simulink model "idc2ff_digital"  (Simulink 8.6)
settings: Solver=ode45  StartTime=0.0  StopTime=10.0  RelTol=1e-3
undefined symbols (not defined in the file or in its folder): M, OSR, tclk
settings Model: Creator=chench  LastModifiedBy=derek
settings OptimizationCC: InitFltsAndDblsToZero=on
settings DebuggingCC: SaveWithParameterizedLinksMsg=none  SignalResolutionControl=TryResolveAllWithWarning  MultiTaskDSMMsg=warning  MultiTaskCondExecSysMsg=none  FcnCallInpInsideContextMsg=UseLocalSettings
settings GRTTargetCC: TargetFcnLib=ansi_tfl_tmw.mat

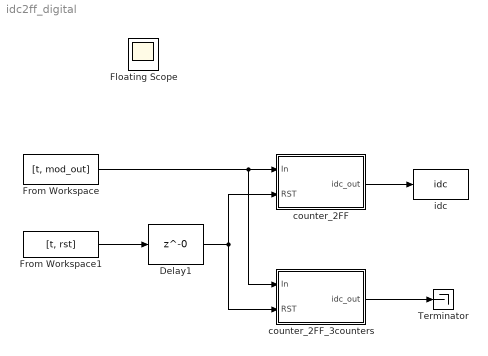
== system idc2ff_digital ==
  Delay1 : Delay  DelayLength=0  InitialCondition=0  InputProcessing=Inherited
  From Workspace : FromWorkspace  VariableName=[t, mod_out]  SampleTime=tclk  Interpolate=off  OutputAfterFinalValue=Holding final value
  From Workspace1 : FromWorkspace  VariableName=[t, rst]  SampleTime=tclk  Interpolate=off  OutputAfterFinalValue=Holding final value
  Terminator : Terminator
  counter_2FF : Subsystem
  counter_2FF_3counters : Subsystem
  idc : ToWorkspace  VariableName=idc  SampleTime=-1
  Floating Scope : Scope
  wires:
  From Workspace/1 -> counter_2FF/1(In), counter_2FF_3counters/1(In)
  counter_2FF/1(idc_out) -> idc/1
  From Workspace1/1 -> Delay1/1
  Delay1/1 -> counter_2FF/2(RST), counter_2FF_3counters/2(RST)
  counter_2FF_3counters/1(idc_out) -> Terminator/1

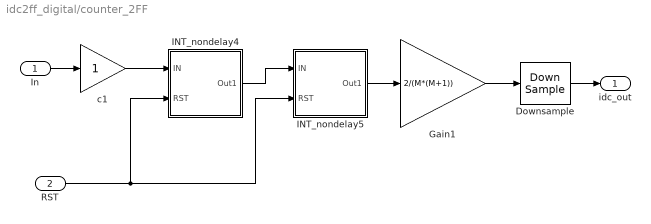
== system idc2ff_digital/counter_2FF ==
  In : Inport
  RST : Inport  Port=2
  Downsample : DownSample  N=OSR  phase=OSR-1  RateOptions=Allow multirate processing
  Gain1 : Gain  Gain=2/(M*(M+1))
  INT_nondelay4 : Subsystem
  INT_nondelay5 : Subsystem
  c1 : Gain  SaturateOnIntegerOverflow=on  OutDataTypeStr=Inherit: Same as input  ParamDataTypeStr=Inherit: Same as input
  idc_out : Outport
  wires:
  RST/1 -> INT_nondelay5/2(RST), INT_nondelay4/2(RST)
  Downsample/1 -> idc_out/1
  c1/1 -> INT_nondelay4/1(IN)
  In/1 -> c1/1
  INT_nondelay4/1(Out1) -> INT_nondelay5/1(IN)
  Gain1/1 -> Downsample/1
  INT_nondelay5/1(Out1) -> Gain1/1

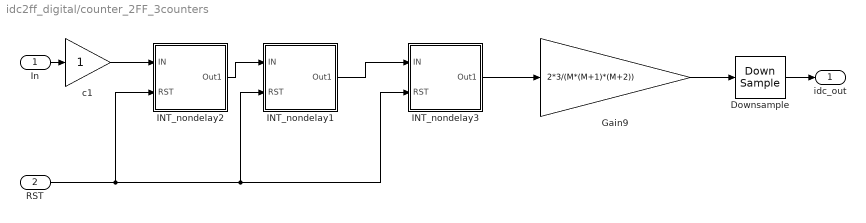
== system idc2ff_digital/counter_2FF_3counters ==
  In : Inport
  RST : Inport  Port=2
  Downsample : DownSample  N=OSR  phase=OSR-1  RateOptions=Allow multirate processing
  Gain9 : Gain  Gain=2*3/(M*(M+1)*(M+2))
  INT_nondelay1 : Subsystem
  INT_nondelay2 : Subsystem
  INT_nondelay3 : Subsystem
  c1 : Gain  SaturateOnIntegerOverflow=on  OutDataTypeStr=Inherit: Same as input  ParamDataTypeStr=Inherit: Same as input
  idc_out : Outport
  wires:
  RST/1 -> INT_nondelay3/2(RST), INT_nondelay1/2(RST), INT_nondelay2/2(RST)
  Downsample/1 -> idc_out/1
  c1/1 -> INT_nondelay2/1(IN)
  In/1 -> c1/1
  INT_nondelay2/1(Out1) -> INT_nondelay1/1(IN)
  INT_nondelay1/1(Out1) -> INT_nondelay3/1(IN)
  INT_nondelay3/1(Out1) -> Gain9/1
  Gain9/1 -> Downsample/1

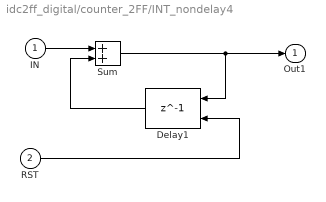
== system idc2ff_digital/counter_2FF/INT_nondelay4 ==
  IN : Inport
  RST : Inport  Port=2
  Delay1 : Delay  DelayLength=1  InitialCondition=0  ExternalReset=Rising  InputProcessing=Inherited
      settings: InputPortMap=u0,r5
  Sum : Sum  SaturateOnIntegerOverflow=on  InputSameDT=on  OutDataTypeStr=Inherit: Same as first input
  Out1 : Outport
  wires:
  IN/1 -> Sum/1
  Sum/1 -> Delay1/1, Out1/1
  RST/1 -> Delay1/2
  Delay1/1 -> Sum/2

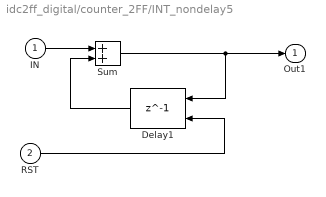
== system idc2ff_digital/counter_2FF/INT_nondelay5 ==
  IN : Inport
  RST : Inport  Port=2
  Delay1 : Delay  DelayLength=1  InitialCondition=0  ExternalReset=Rising  InputProcessing=Inherited
      settings: InputPortMap=u0,r5
  Sum : Sum  SaturateOnIntegerOverflow=on  InputSameDT=on  OutDataTypeStr=Inherit: Same as first input
  Out1 : Outport
  wires:
  IN/1 -> Sum/1
  Sum/1 -> Delay1/1, Out1/1
  RST/1 -> Delay1/2
  Delay1/1 -> Sum/2

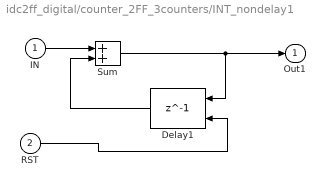
== system idc2ff_digital/counter_2FF_3counters/INT_nondelay1 ==
  IN : Inport
  RST : Inport  Port=2
  Delay1 : Delay  DelayLength=1  InitialCondition=0  ExternalReset=Rising  InputProcessing=Inherited
      settings: InputPortMap=u0,r5
  Sum : Sum  SaturateOnIntegerOverflow=on  InputSameDT=on  OutDataTypeStr=Inherit: Same as first input
  Out1 : Outport
  wires:
  IN/1 -> Sum/1
  Sum/1 -> Delay1/1, Out1/1
  RST/1 -> Delay1/2
  Delay1/1 -> Sum/2

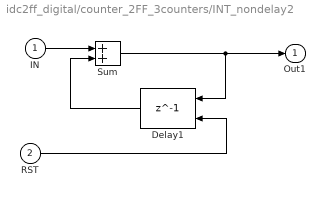
== system idc2ff_digital/counter_2FF_3counters/INT_nondelay2 ==
  IN : Inport
  RST : Inport  Port=2
  Delay1 : Delay  DelayLength=1  InitialCondition=0  ExternalReset=Rising  InputProcessing=Inherited
      settings: InputPortMap=u0,r5
  Sum : Sum  SaturateOnIntegerOverflow=on  InputSameDT=on  OutDataTypeStr=Inherit: Same as first input
  Out1 : Outport
  wires:
  IN/1 -> Sum/1
  Sum/1 -> Delay1/1, Out1/1
  RST/1 -> Delay1/2
  Delay1/1 -> Sum/2

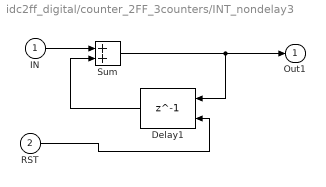
== system idc2ff_digital/counter_2FF_3counters/INT_nondelay3 ==
  IN : Inport
  RST : Inport  Port=2
  Delay1 : Delay  DelayLength=1  InitialCondition=0  ExternalReset=Rising  InputProcessing=Inherited
      settings: InputPortMap=u0,r5
  Sum : Sum  SaturateOnIntegerOverflow=on  InputSameDT=on  OutDataTypeStr=Inherit: Same as first input
  Out1 : Outport
  wires:
  IN/1 -> Sum/1
  Sum/1 -> Delay1/1, Out1/1
  RST/1 -> Delay1/2
  Delay1/1 -> Sum/2
